simulink model "Project_Architecture"  (R2025b)
settings: Solver=FixedStepAuto  StartTime=0.0  StopTime=200  FixedStep=0.1  RelTol=1e-3
values from neighbouring files (symbols this model uses):
  A = [0.00, 0.30, 0.40, 0.30 ... (first row only)    [init_params.m]
  A_row_sum = sum(A, 2)    [init_params.m]
  b = [0.30; 0.20; 0.50; 0.40]    [init_params.m]
  c = [9.00; 7.00; 11.00; 7.00]    [init_params.m]
  dif_val = dif    [init_params.m]
  get_val = get    [init_params.m]
  off_val = off    [init_params.m]
  on_val = on    [init_params.m]
  u_temp = 6    [init_params.m]
  x0 = [16.5; 16.5; 16.5; 16.5]    [init_params.m]
settings Model: Creator=My NoteBook  LastModifiedBy=My NoteBook
settings SolverCC: AutoInsertRateTranBlk=on
settings OptimizationCC: EnhancedBackFolding=on  PassReuseOutputArgsAs=Individual arguments  ZeroExternalMemoryAtStartup=off  ZeroInternalMemoryAtStartup=off  MaxStackSize=64  OptimizeBlockOrder=speed  DifferentSizesBufferReuse=on  OptimizationCustomize=off  EfficientTunableParamExpr=on
settings DebuggingCC: ParameterTunabilityLossMsg=error
settings HardwareCC: ProdBitPerInt=16.0  ProdBitPerPointer=16.0  ProdBitPerSizeT=16.0  ProdBitPerPtrDiffT=16.0  ProdLargestAtomicFloat=None  ProdWordSize=8.0  ProdHWDeviceType=Atmel->AVR
settings SFSimCC: MATLABDynamicMemAlloc=off
settings RTWCC: SystemTargetFile=ert.tlc  TemplateMakefile=ert_default_tmf  Toolchain=Arduino AVR  BuildConfiguration=Faster Runs  Description=Embedded Coder
settings CodeAppCC: ForceParamTrailComments=on  IgnoreCustomStorageClasses=off  OperatorAnnotations=on  SimulinkDataObjDesc=on  SFDataObjDesc=on  InsertBlockDesc=on
settings ERTTargetCC: ExtModeTransport=3.0  ExtModeStaticAlloc=on  ExtModeStaticAllocSize=250.0  ExtModeMexFile=ext_xcp  ExtModeIntrfLevel=Level2 - Open  InlinedParameterPlacement=Hierarchical  ERTCustomFileTemplate=example_file_process.tlc  SupportContinuousTime=on

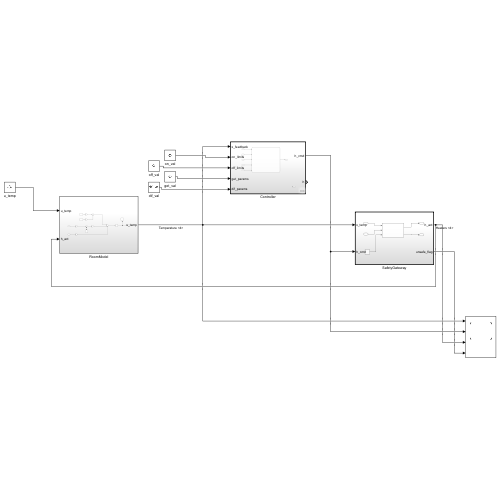
[thumbnail: Simulink's stored preview of the top-level diagram]
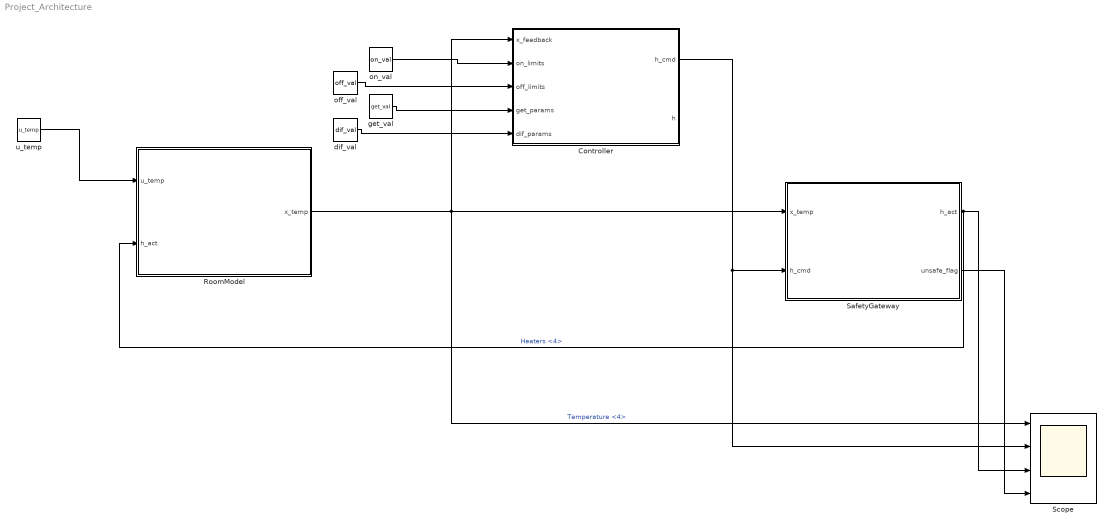
== system Project_Architecture ==
  Controller : Subsystem  TreatAsAtomicUnit=on  SystemSampleTime=0.1
  RoomModel : Subsystem
  SafetyGateway : Subsystem  TreatAsAtomicUnit=on  SystemSampleTime=0.1
  Scope : Scope  NumInputPorts=4
      settings: ActiveDisplayYMinimum=-3.0766030509506344  ActiveDisplayYMaximum=23.862152939436026
  dif_val : Constant  Value=dif_val
  get_val : Constant  Value=get_val
  off_val : Constant  Value=off_val
  on_val : Constant  Value=on_val
  u_temp : Constant  Value=u_temp
  wires:
  u_temp/1 -> RoomModel/1(u_temp)
  SafetyGateway/1(h_act) -> RoomModel/2(h_act), Scope/3  "Heaters <4>"
  RoomModel/1(x_temp) -> Scope/1, SafetyGateway/1(x_temp), Controller/1(x_feedback)  "Temperature <4>"
  Controller/1(h_cmd) -> SafetyGateway/2(h_cmd), Scope/2
  SafetyGateway/2(unsafe_flag) -> Scope/4
  on_val/1 -> Controller/2(on_limits)
  off_val/1 -> Controller/3(off_limits)
  get_val/1 -> Controller/4(get_params)
  dif_val/1 -> Controller/5(dif_params)

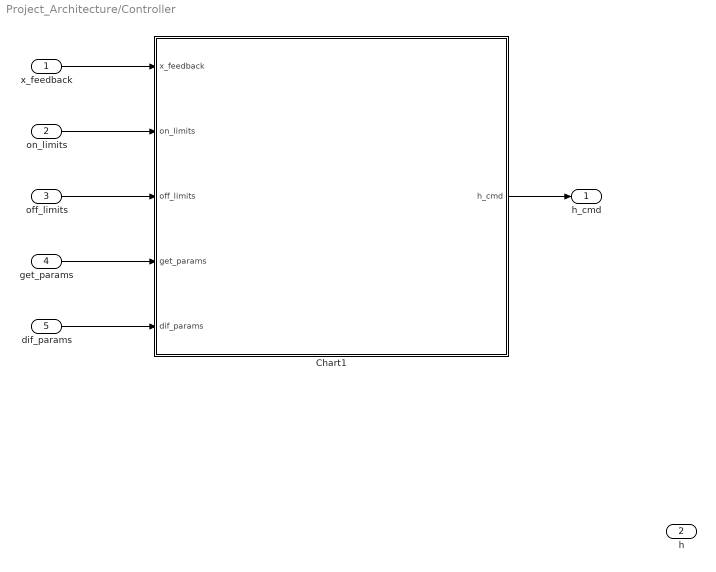
== system Project_Architecture/Controller ==
  x_feedback : Inport
  on_limits : Inport  Port=2
  off_limits : Inport  Port=3
  get_params : Inport  Port=4
  dif_params : Inport  Port=5
  Chart1 : Stateflow chart  TreatAsAtomicUnit=on
  h_cmd : Outport
  h : Outport  Port=2
  wires:
  x_feedback/1 -> Chart1/1(x_feedback)
  Chart1/1(h_cmd) -> h_cmd/1
  off_limits/1 -> Chart1/3(off_limits)
  get_params/1 -> Chart1/4(get_params)
  dif_params/1 -> Chart1/5(dif_params)
  on_limits/1 -> Chart1/2(on_limits)

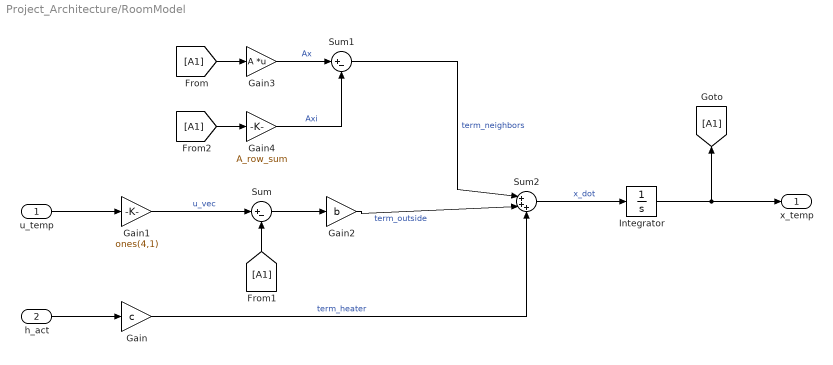
== system Project_Architecture/RoomModel ==
  u_temp : Inport  PortDimensions=1
  h_act : Inport  Port=2  PortDimensions=4
  Gain : Gain  Gain=c
  Gain1 : Gain  Gain=ones(4,1)
  Gain2 : Gain  Gain=b
  Gain3 : Gain  Gain=A  Multiplication=Matrix(K*u)
  Gain4 : Gain  Gain=A_row_sum
  Integrator : Integrator  InitialCondition=x0
  Sum : Sum  Inputs=|+-
  Sum1 : Sum  Inputs=|+-
  Sum2 : Sum  Inputs=|+++
  x_temp : Outport  PortDimensions=4
  wires:
  u_temp/1 -> Gain1/1
  h_act/1 -> Gain/1
  Gain/1 -> Sum2/3  "term_heater"
  Gain1/1 -> Sum/1  "u_vec"
  Sum/1 -> Gain2/1
  Gain4/1 -> Sum1/2  "Axi"
  Gain3/1 -> Sum1/1  "Ax"
  Sum1/1 -> Sum2/1  "term_neighbors"
  Gain2/1 -> Sum2/2  "term_outside"
  Sum2/1 -> Integrator/1  "x_dot"
  Integrator/1 -> x_temp/1, [A1]
  [A1] -> Gain3/1
  [A1] -> Sum/2
  [A1] -> Gain4/1

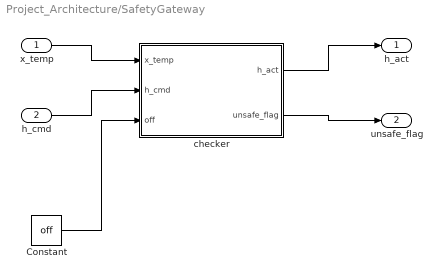
== system Project_Architecture/SafetyGateway ==
  x_temp : Inport  PortDimensions=4
  h_cmd : Inport  Port=2  PortDimensions=4
  Constant : Constant  Value=off
  checker : MATLAB Function  TreatAsAtomicUnit=on
  h_act : Outport  PortDimensions=4
  unsafe_flag : Outport  Port=2  PortDimensions=1
  wires:
  x_temp/1 -> checker/1(x_temp)
  h_cmd/1 -> checker/2(h_cmd)
  checker/1(h_act) -> h_act/1
  checker/2(unsafe_flag) -> unsafe_flag/1
  Constant/1 -> checker/3(off)

== matlab function Project_Architecture/SafetyGateway/checker ==
  data: x_temp input size=4; h_act output size=4; h_cmd input size=4; unsafe_flag output size=1; off input
function [h_act, unsafe_flag] = checker(x_temp, h_cmd, off)

persistent h_prev
if isempty(h_prev)
    h_prev = zeros(4,1);
end

unsafe_flag = 0;

% Force column vectors
x = x_temp(:);
h = h_cmd(:);

h_rounded = round(h);

if any(abs(h - h_rounded) > 1e-6)
    unsafe_flag = 1;
    h_act = h_prev;
    return;
end

h = h_rounded;

if sum(h) > 2
    unsafe_flag = 1;
    h_act = h_prev;
    return;
end

for i = 1:4
    if x(i) >= off(i) && h(i) == 1
        unsafe_flag = 1;
        h_act = h_prev;
        return;
    end
end

h_act = h;
h_prev = h_act;

== stateflow chart Project_Architecture/Controller/Chart1 ==
  settings: sampleTime=0.01
  state S1100
    state S3
    (default) -> S1100.S3
    S1100.S3 -> S1100.S3 [order 4] : [x_feedback(2)>=off_limits(2) && h_cmd(2) == 1]{h_cmd(2) = 0;}
    S1100.S3 -> S1100.S3 [order 3] : [x_feedback(2) <=on_limits(2) && h_cmd(2) == 0]{h_cmd(2) = 1;}
    S1100.S3 -> S1100.S3 [order 2] : [x_feedback(1) <=on_limits(1) && h_cmd(1) == 0]{h_cmd(1) = 1;}
    S1100.S3 -> S1100.S3 [order 1] : [x_feedback(1)>=off_limits(1) && h_cmd(1) == 1]{h_cmd(1) = 0;}
  state S0110
    state S3
    (default) -> S0110.S3
    S0110.S3 -> S0110.S3 [order 4] : [x_feedback(2)>=off_limits(2) && h_cmd(2) == 1]{h_cmd(2) = 0;}
    S0110.S3 -> S0110.S3 [order 3] : [x_feedback(2) <=on_limits(2) && h_cmd(2) == 0]{h_cmd(2) = 1;}
    S0110.S3 -> S0110.S3 [order 2] : [x_feedback(3) <=on_limits(3) && h_cmd(3) == 0]{h_cmd(3) = 1;}
    S0110.S3 -> S0110.S3 [order 1] : [x_feedback(3)>=off_limits(3) && h_cmd(3) == 1]{h_cmd(3) = 0;}
  state S0101
    state S3
    (default) -> S0101.S3
    S0101.S3 -> S0101.S3 [order 4] : [x_feedback(2)>=off_limits(2) && h_cmd(2) == 1]{h_cmd(2) = 0;}
    S0101.S3 -> S0101.S3 [order 3] : [x_feedback(2) <=on_limits(2) && h_cmd(2) == 0]{h_cmd(2) = 1;}
    S0101.S3 -> S0101.S3 [order 2] : [x_feedback(4) <=on_limits(4) && h_cmd(4) == 0]{h_cmd(4) = 1;}
    S0101.S3 -> S0101.S3 [order 1] : [x_feedback(4)>=off_limits(4) && h_cmd(4) == 1]{h_cmd(4) = 0;}
  state S0011
    state S3
    S0011.S3 -> S0011.S3 [order 4] : [x_feedback(4)>=off_limits(4) && h_cmd(4) == 1]{h_cmd(4) = 0;}
    S0011.S3 -> S0011.S3 [order 3] : [x_feedback(4) <=on_limits(4) && h_cmd(4) == 0]{h_cmd(4) = 1;}
    S0011.S3 -> S0011.S3 [order 2] : [x_feedback(3) <=on_limits(3) && h_cmd(3) == 0]{h_cmd(3) = 1;}
    S0011.S3 -> S0011.S3 [order 1] : [x_feedback(3)>=off_limits(3) && h_cmd(3) == 1]{h_cmd(3) = 0;}
  state S1001
    state S3
    (default) -> S1001.S3
    S1001.S3 -> S1001.S3 [order 2] : [x_feedback(4)>=off_limits(4) && h_cmd(4) == 1]{h_cmd(4) = 0;}
    S1001.S3 -> S1001.S3 [order 1] : [x_feedback(4) <=on_limits(4) && h_cmd(4) == 0]{h_cmd(4) = 1;}
    S1001.S3 -> S1001.S3 [order 4] : [x_feedback(1) <=on_limits(1) && h_cmd(1) == 0]{h_cmd(1) = 1;}
    S1001.S3 -> S1001.S3 [order 3] : [x_feedback(1)>=off_limits(1) && h_cmd(1) == 1]{h_cmd(1) = 0;}
  state S1010
    state S3
    (default) -> S1010.S3
    S1010.S3 -> S1010.S3 [order 4] : [x_feedback(3)>=off_limits(3) && h_cmd(3) == 1]{h_cmd(3) = 0;}
    S1010.S3 -> S1010.S3 [order 3] : [x_feedback(3) <=on_limits(3) && h_cmd(3) == 0]{h_cmd(3) = 1;}
    S1010.S3 -> S1010.S3 [order 2] : [x_feedback(1) <=on_limits(1) && h_cmd(1) == 0]{h_cmd(1) = 1;}
    S1010.S3 -> S1010.S3 [order 1] : [x_feedback(1)>=off_limits(1) && h_cmd(1) == 1]{h_cmd(1) = 0;}
  (default) -> S0110 [order 1]
  S0110 -> S1100 [order 1] : [x_feedback(1) <=get_params(1) && x_feedback(3) - x_feedback(1) >= dif_params(1)]{h_cmd(3) = 0; h_cmd(1) = 1;}
  S1100 -> S0110 [order 1] : [x_feedback(3) <=get_params(3) && x_feedback(1) - x_feedback(3) >= dif_params(3)]{h_cmd(1) = 0; h_cmd(3) = 1;}
  S1001 -> S1100 [order 4] : [x_feedback(2) <=get_params(2) && x_feedback(4) - x_feedback(2) >= dif_params(2)]{h_cmd(4) = 0; h_cmd(2) = 1;}
  S0110 -> S1010 [order 3] : [x_feedback(1) <=get_params(1) && x_feedback(2) - x_feedback(1) >= dif_params(1)]{h_cmd(2) = 0; h_cmd(1) = 1;}
  S1100 -> S1001 [order 3] : [x_feedback(4) <=get_params(4) && x_feedback(2) - x_feedback(4) >= dif_params(4)]{h_cmd(2) = 0; h_cmd(4) = 1;}
  S0101 -> S0110 [order 1] : [x_feedback(3) <=get_params(3) && x_feedback(4) - x_feedback(3) >= dif_params(3)]{h_cmd(4) = 0; h_cmd(3) = 1;}
  S1010 -> S0110 [order 1] : [x_feedback(2) <=get_params(2) && x_feedback(1) - x_feedback(2) >= dif_params(2)]{h_cmd(1) = 0; h_cmd(2) = 1;}
  S1010 -> S1100 [order 4] : [x_feedback(2) <=get_params(2) && x_feedback(3) - x_feedback(2) >= dif_params(2)]{h_cmd(3) = 0; h_cmd(2) = 1;}
  S1100 -> S0101 [order 2] : [x_feedback(4) <=get_params(4) && x_feedback(1) - x_feedback(4) >= dif_params(4)]{h_cmd(1) = 0; h_cmd(4) = 1;}
  S0101 -> S1100 [order 2] : [x_feedback(1) <=get_params(1) && x_feedback(4) - x_feedback(1) >= dif_params(1)]{h_cmd(4) = 0; h_cmd(1) = 1;}
  S0110 -> S0101 [order 2] : [x_feedback(4) <=get_params(4) && x_feedback(3) - x_feedback(4) >= dif_params(4)]{h_cmd(3) = 0; h_cmd(4) = 1;}
  (default) -> S1010 [order 3] : [x_feedback(3) <=get_params(3) && x_feedback(2) - x_feedback(3) >= dif_params(3)]{h_cmd(2) = 0; h_cmd(3) = 1;}
  S0011 -> S0110 [order 1] : [x_feedback(2) <=get_params(2) && x_feedback(4) - x_feedback(2) >= dif_params(2)]{h_cmd(4) = 0; h_cmd(2) = 1;}
  S0110 -> S0011 [order 4] : [x_feedback(4) <=get_params(4) && x_feedback(2) - x_feedback(4) >= dif_params(4)]{h_cmd(2) = 0; h_cmd(4) = 1;}
  (default) -> S0011.S3 [order 2]
  S0011 -> S0101 [order 3] : [x_feedback(2) <=get_params(2) && x_feedback(3) - x_feedback(2) >= dif_params(2)]{h_cmd(3) = 0; h_cmd(2) = 1;}
  S0101 -> S0011 [order 4] : [x_feedback(3) <=get_params(3) && x_feedback(2) - x_feedback(3) >= dif_params(3)]{h_cmd(2) = 0; h_cmd(3) = 1;}
  S1001 -> S0011 [order 1] : [x_feedback(3) <=get_params(3) && x_feedback(1) - x_feedback(3) >= dif_params(3)]{h_cmd(1) = 0; h_cmd(3) = 1;}
  S0011 -> S1001 [order 4] : [x_feedback(1) <=get_params(1) && x_feedback(3) - x_feedback(1) >= dif_params(1)]{h_cmd(3) = 0; h_cmd(1) = 1;}
  S0101 -> S1001 [order 3] : [x_feedback(1) <=get_params(1) && x_feedback(2) - x_feedback(1) >= dif_params(1)]{h_cmd(2) = 0; h_cmd(1) = 1;}
  S1001 -> S0101 [order 2] : [x_feedback(2) <=get_params(2) && x_feedback(1) - x_feedback(2) >= dif_params(2)]{h_cmd(1) = 0; h_cmd(2) = 1;}
  S1010 -> S0011 [order 2] : [x_feedback(4) <=get_params(4) && x_feedback(1) - x_feedback(4) >= dif_params(4)]{h_cmd(1) = 0; h_cmd(4) = 1;}
  S0011 -> S1010 [order 2] : [x_feedback(1) <=get_params(1) && x_feedback(4) - x_feedback(1) >= dif_params(1)]{h_cmd(4) = 0; h_cmd(1) = 1;}
  S1001 -> S1010 [order 3] : [x_feedback(3) <=get_params(3) && x_feedback(4) - x_feedback(3) >= dif_params(3)]{h_cmd(4) = 0; h_cmd(3) = 1;}
  S1010 -> S1001 [order 3] : [x_feedback(4) <=get_params(4) && x_feedback(3) - x_feedback(4) >= dif_params(4)]{h_cmd(3) = 0; h_cmd(4) = 1;}
  data: x_feedback input size=[1 4]; h_cmd output size=[1 4] =[0 1 1 0]; on_limits input size=[1 4]; off_limits input size=[1 4]; get_params input size=[1 4]; dif_params input size=[1 4]
